simulink model "cuk_switched_equation_model"  (R2023b)
settings: Solver=ode4  StartTime=0.0  StopTime=0.02  FixedStep=Ts/200  RelTol=1e-3
undefined symbols (not defined in the file or in its folder): C1, Co, D, ESR, I1_init, I2_init, L1, L2, Rload, Ts, VC_init, Vin, VO_init
settings Model: Creator=ZLM  LastModifiedBy=ZLM

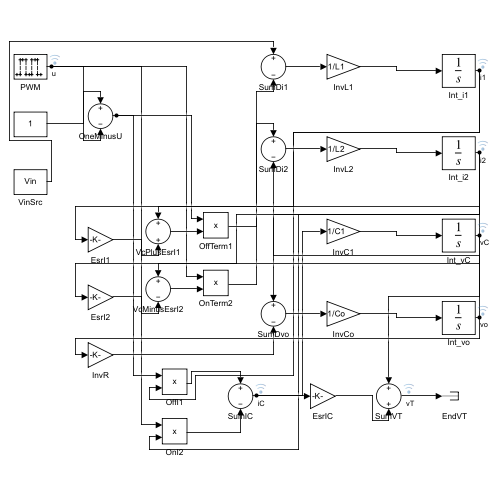
[thumbnail: Simulink's stored preview of the top-level diagram]
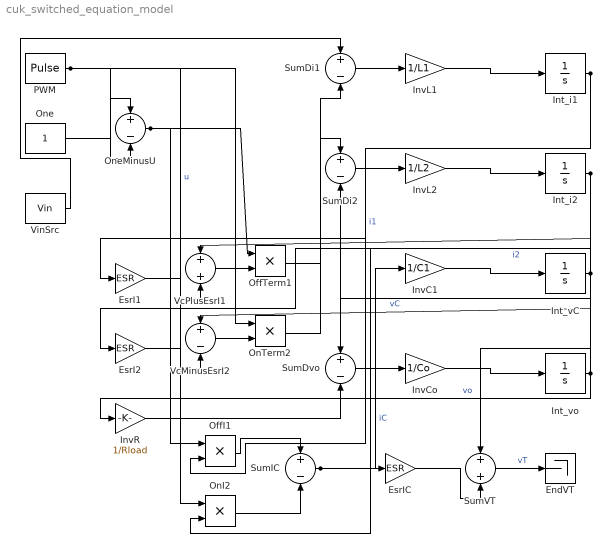
== system cuk_switched_equation_model ==
  EndVT : Terminator
  EsrI1 : Gain  Gain=ESR
  EsrI2 : Gain  Gain=ESR
  EsrIC : Gain  Gain=ESR
  Int_i1 : Integrator  InitialCondition=I1_init
  Int_i2 : Integrator  InitialCondition=I2_init
  Int_vC : Integrator  InitialCondition=VC_init
  Int_vo : Integrator  InitialCondition=VO_init
  InvC1 : Gain  Gain=1/C1
  InvCo : Gain  Gain=1/Co
  InvL1 : Gain  Gain=1/L1
  InvL2 : Gain  Gain=1/L2
  InvR : Gain  Gain=1/Rload
  OffI1 : Product
  OffTerm1 : Product
  OnI2 : Product
  OnTerm2 : Product
  One : Constant
  OneMinusU : Sum  Inputs=+-
  PWM : DiscretePulseGenerator  Period=200  PulseWidth=round(200*D)  SampleTime=Ts/200
  SumDi1 : Sum  Inputs=+-
  SumDi2 : Sum  Inputs=+-
  SumDvo : Sum  Inputs=+-
  SumIC : Sum  Inputs=+-
  SumVT : Sum
  VcMinusEsrI2 : Sum  Inputs=+-
  VcPlusEsrI1 : Sum
  VinSrc : Constant  Value=Vin
  wires:
  PWM/1 -> OneMinusU/2, OnI2/1, OnTerm2/1  "u"
  One/1 -> OneMinusU/1
  OneMinusU/1 -> OffI1/1, OffTerm1/1
  Int_i1/1 -> OffI1/2, EsrI1/1  "i1"
  Int_i2/1 -> OnI2/2, EsrI2/1, SumDvo/1  "i2"
  OffI1/1 -> SumIC/1
  OnI2/1 -> SumIC/2
  Int_vC/1 -> VcPlusEsrI1/1, VcMinusEsrI2/1, SumVT/1  "vC"
  EsrI1/1 -> VcPlusEsrI1/2
  VcPlusEsrI1/1 -> OffTerm1/2
  VinSrc/1 -> SumDi1/1
  OffTerm1/1 -> SumDi1/2
  SumDi1/1 -> InvL1/1
  InvL1/1 -> Int_i1/1
  EsrI2/1 -> VcMinusEsrI2/2
  VcMinusEsrI2/1 -> OnTerm2/2
  OnTerm2/1 -> SumDi2/1
  Int_vo/1 -> SumDi2/2, InvR/1  "vo"
  SumDi2/1 -> InvL2/1
  InvL2/1 -> Int_i2/1
  SumIC/1 -> InvC1/1, EsrIC/1  "iC"
  InvC1/1 -> Int_vC/1
  InvR/1 -> SumDvo/2
  SumDvo/1 -> InvCo/1
  InvCo/1 -> Int_vo/1
  EsrIC/1 -> SumVT/2
  SumVT/1 -> EndVT/1  "vT"
